simulink model "sample"  (R2017a)
settings: Solver=VariableStepAuto  StartTime=0.0  StopTime=10.0  RelTol=1e-3
libraries: dsparch4 x2
settings Model: Creator=zfb15  LastModifiedBy=zfb15

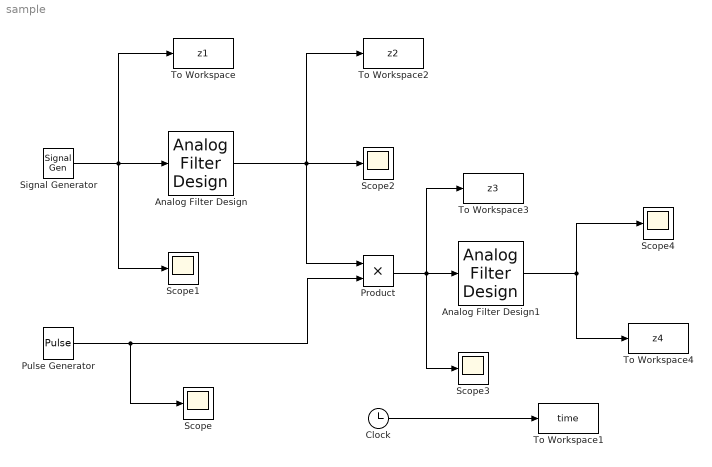
== system sample ==
  Analog Filter Design : dsparch4/Analog Filter Design  method=Butterworth  filttype=Lowpass  N=8  Wlo=62800  Whi=80  Rp=2  Rs=40
  Analog Filter Design1 : dsparch4/Analog Filter Design  method=Butterworth  filttype=Lowpass  N=8  Wlo=25132  Whi=80  Rp=2  Rs=40
  Clock : Clock
  Product : Product
  Pulse Generator : DiscretePulseGenerator  PulseType=Time based  Period=0.0003  PulseWidth=50
  Scope{,1..4} (5 alike) : Scope
  Signal Generator : SignalGenerator  Amplitude=2  Frequency=2000
  To Workspace : ToWorkspace  VariableName=z1  SampleTime=-1
  To Workspace1 : ToWorkspace  VariableName=time  SampleTime=-1
  To Workspace2 : ToWorkspace  VariableName=z2  SampleTime=-1
  To Workspace3 : ToWorkspace  VariableName=z3  SampleTime=-1
  To Workspace4 : ToWorkspace  VariableName=z4  SampleTime=-1
  wires:
  Signal Generator/1 -> Scope1/1, To Workspace/1, Analog Filter Design/1
  Pulse Generator/1 -> Product/2, Scope/1
  Clock/1 -> To Workspace1/1
  Analog Filter Design/1 -> Product/1, To Workspace2/1, Scope2/1
  Product/1 -> To Workspace3/1, Analog Filter Design1/1, Scope3/1
  Analog Filter Design1/1 -> To Workspace4/1, Scope4/1
